simulink library "Fan_Const"  (R2018b)
settings: Solver=VariableStepAuto  StartTime=0.0  StopTime=10.0  RelTol=1e-3
undefined symbols (not defined in the file): density
libraries: carnot x1
settings Model: Creator=drhf  LastModifiedBy=drhf

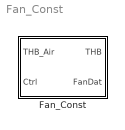
== system Fan_Const ==
  Fan_Const : Subsystem  mask(Fan constant){Vdotmax=1000, dia=0.5, p0=101300, mix=0.01, Tini=20, UA=3, mcp=1000, e0=10, e1=10, e2=-1}
      mask prompts: Vdotmax "Vdotmax : volume flowrate in m³/h"; dia "diameter at in- and outlet [m]"; p0 "air pressure in Pa"; mix "kg of water per kg of dry air"; Tini "ambient and start temperature in °C"; UA "Thermal loss coefficient to ambient in W/K"; mcp "mcp: thermal capacity of the node in J/K"; e0 "e0: constant coefficient in W"; e1 "e1: linear coefficient in W*s/kg"; e2 "e2: quadratic coefficient in W*(s/kg)²"
      mask help:
      | Model of a fan for air ventilation systems. Volume flowrate is constant according to the parameter Vdotmax and the control signal:
      | Vdot = Vdotmax * Ctrl
      | Keep in mind that the flowrate in the THB is the massflowrate in kg/s whereas the parameters of the fan have different units.
      | mdot = Vdot/3600 * density(Tamb, air_pressure, FluidAir, kgH2O/kgAir)
      | Use the option "thermal node" if you want the pump to have thermal capacity and losses to ambient (or if you want to break an algebraic loop in the temperature signal).
      | Electric power is calculated Pel = e0 + e1*mdot + e2*mdot^2
      mask Help: web(fullfile(path_carnot('help'),'Fan_Const.html'),'-helpbrowser')
      mask TypeOptions dia: Pump_Const/dia
      mask TypeOptions mix: Pump_Const/mix
      mask TypeOptions Tini: Pump_Const/Tini
      mask TypeOptions UA: Pump_Const/UA
      mask TypeOptions mcp: Pump_Const/mcp
      mask TypeOptions e0: Pump_Const/e0
      mask TypeOptions e1: Pump_Const/e1
      mask TypeOptions e2: Pump_Const/e2
      mask DialogControl ParameterTabVar0 Prompt: Hydraulic
      mask DialogControl Container7 Prompt: Initial Values
      mask DialogControl ParameterTabVar012 Prompt: Thermal
      mask DialogControl ParameterTabVar01 Prompt: Electric
      mask Display:
      | plot(-40,-20,130,100, ...
      |     [0,0,10,30,50,70,80,80,70,50,30,10,0],[50,30,10,0,0,10,30,50,70,80,80,70,50], ...
      |     [80,10],[50,70], ...
      |     [80,10],[30,10])

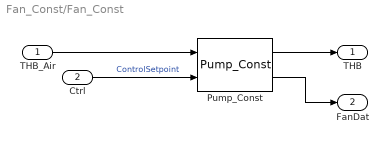
== system Fan_Const/Fan_Const ==
  THB_Air : Inport
  Ctrl : Inport  Port=2
  Pump_Const : carnot/Hydraulics/Pump_Const  mdotmax=Vdotmax/3600*density(Tini,p0,2,0)  dia=dia  p0=p0  fluid_id=Air  mix=mix  mix2=0  mix3=0  UA=UA  mcp=mcp  Tini=Tini  e0=e0  e1=e1  e2=e2
      settings: SourceProductName=Carnot
  THB : Outport
  FanDat : Outport  Port=2
  wires:
  THB_Air/1 -> Pump_Const/1
  Ctrl/1 -> Pump_Const/2  "ControlSetpoint"
  Pump_Const/1 -> THB/1
  Pump_Const/2 -> FanDat/1
